simulink model "GPCA_LoggingNoActions"  (Simulink 9.0)
settings: Solver=VariableStepAuto  StartTime=0.0  StopTime=10.0  RelTol=1e-3  EnableMultiTasking=on
settings Model: SuppressorTable=22 serialization::archive 11 0 6 0 0 0 0 0  Creator=bourbouh  LastModifiedBy=ktrinh
settings DataIOCC: SaveFormat=Dataset
settings DebuggingCC: UnderspecifiedInitializationDetection=Simplified  MergeDetectMultiDrivingBlocksExec=error
settings HardwareCC: ProdBitPerPointer=64  ProdBitPerSizeT=64  ProdBitPerPtrDiffT=64  ProdLargestAtomicFloat=Float  ProdIntDivRoundTo=Zero  ProdEndianess=LittleEndian  ProdWordSize=64  ProdHWDeviceType=Intel->x86-64 (Windows64)
settings ModelReferenceCC: PropagateSignalLabelsOutOfModel=on
settings GRTTargetCC: GeneratePreprocessorConditionals=Disable all

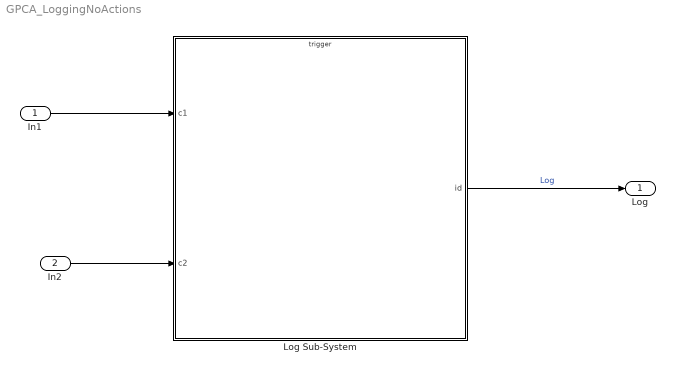
== system GPCA_LoggingNoActions ==
  In1 : Inport  OutDataTypeStr=boolean
  In2 : Inport  Port=2  OutDataTypeStr=boolean
  Log Sub-System : Stateflow chart  TreatAsAtomicUnit=on
  Log : Outport
  wires:
  Log Sub-System/1(id) -> Log/1  "Log"
  In1/1 -> Log Sub-System/1(c1)
  In2/1 -> Log Sub-System/2(c2)

== stateflow chart Log Sub-System ==
  state NOT_ON
    entry: id = 1;
  state LOG
    entry: id=2;
  (default) -> NOT_ON [order 2]
  (default) -> LOG [order 1] : c0
  NOT_ON -> LOG : [c1]
  LOG -> NOT_ON : [c2]
  data: c1 input boolean; c2 input boolean; id output double
  events: c0 input RISING_EDGE_EVENT
